simulink model "variense_block"  (R2018b)
settings: Solver=FixedStepDiscrete  StartTime=0.0  StopTime=inf  FixedStep=.0001  RelTol=1e-3
InitFcn:
  | addpath('..\ForceSensor\compile\release')
libraries: xpcutilitieslib x6, etargetslib x4, aerolibanimutils x1
settings Model: Creator=dds  LastModifiedBy=dds

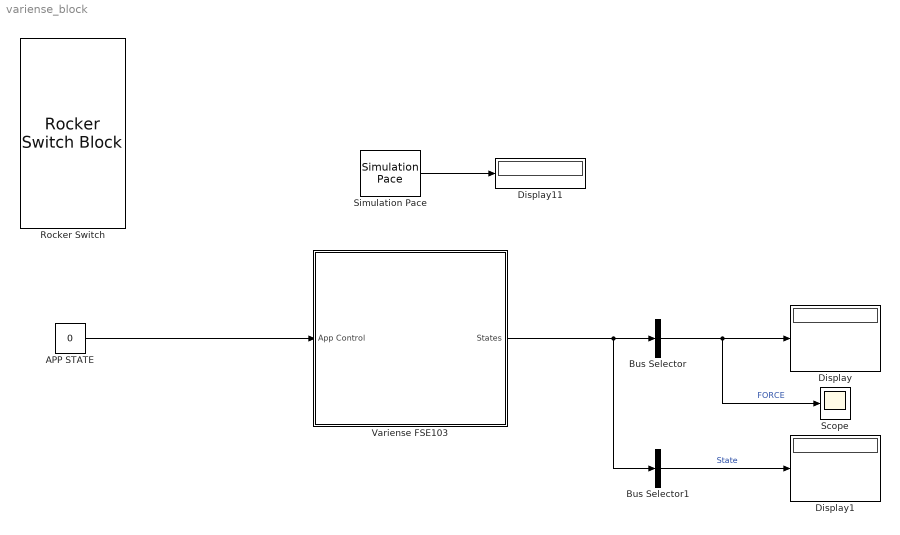
== system variense_block ==
  APP STATE : Constant  Value=0  OutDataTypeStr=uint32
  Bus Selector : BusSelector  OutputSignals=Fx,Fy,Fz  OutputAsBus=on
  Bus Selector1 : BusSelector  OutputSignals=Reception Rate [us],Packets received  OutputAsBus=on
  Display : Display
  Display1 : Display
  Display11 : Display
  Rocker Switch : RockerSwitchBlock  WebBlockId=99
      settings: Values={{'STOP', 'START'}, [1 0]}
  Scope : Scope
  Simulation Pace : aerolibanimutils/Simulation Pace  SimulationPace=1  SleepMode=Auto  OutputPaceError=on  SampleTime=-1
  "Variense FSE103 " : Subsystem  mask{id=1, port='COM8', baudrate=10.5Mbps, ts=1, reg_name='DefenceRobot', reg_size=512, st=0}
      mask prompts: id "Sensor Id"; ts "Sample Time [us]"; reg_name "Register Name"; reg_size "Register Size"; st "Start address"
      mask TypeOptions baudrate: 9600 btps | 57600 bps | 115200 bps | 1 Mbps | 2 Mbps | 3 Mbps | 4 Mbps | 4.5 Mbps | 10.5Mbps
      mask DialogControl DescGroupVar Prompt: IApp based Block
      mask DialogControl Container4 Prompt: Device Control Parameters
      mask DialogControl Container6 Prompt: Main Register Parameters
      mask Display:
      | image('variense.jpg')
      | color('red');
      | 
      | port_label('output', 1, 'Sensors' )
      | color('blue');
      | port_label('input', 1, 'App Control')
  wires:
  Simulation Pace/1 -> Display11/1
  APP STATE/1 -> "Variense FSE103 "/1(App Control)
  "Variense FSE103 "/1(States) -> Bus Selector1/1, Bus Selector/1
  Bus Selector/1 -> Scope/1, Display/1  "FORCE"
  Bus Selector1/1 -> Display1/1  "State"

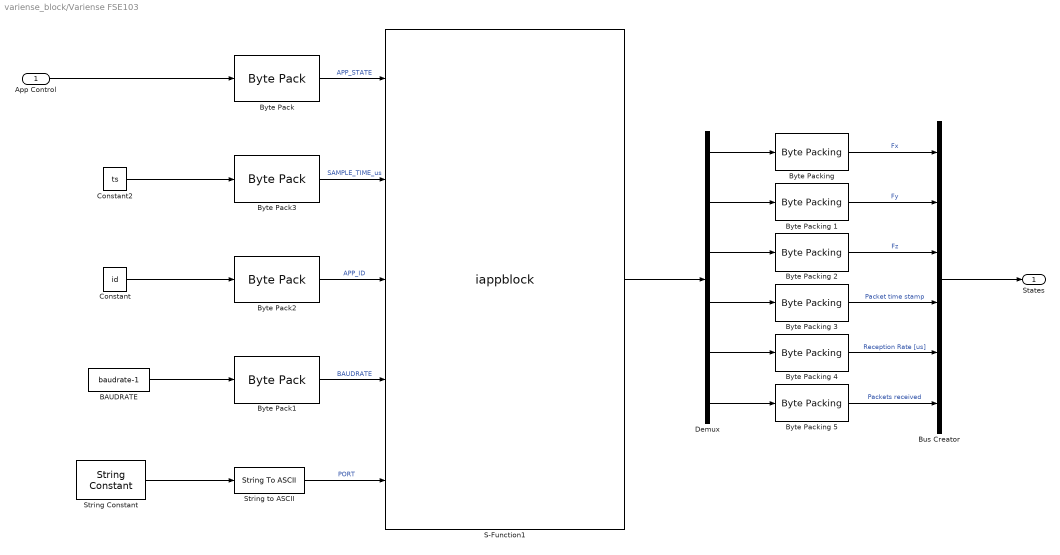
== system variense_block/Variense FSE103  ==
  App Control : Inport
  BAUDRATE : Constant  Value=baudrate-1  OutDataTypeStr=uint32
  Bus Creator : BusCreator  Inputs=6
  Byte Pack{,1..3} (4 alike) : etargetslib/Byte Pack  datatypes={'uint32'}  byteAlign=1
  Byte Packing {,1..5} (6 alike) : xpcutilitieslib/Byte Packing 
  Constant : Constant  Value=id  OutDataTypeStr=uint32
  Constant2 : Constant  Value=ts  OutDataTypeStr=uint32
  Demux : Demux  Outputs=6
  S-Function1 : S-Function  FunctionName=iappblock  Parameters=configText,prog,ts,trig,cmd  SFunctionDeploymentMode=off  EnableBusSupport=off  mask{configText=|, prog=which('ForceSensor.exe'), ts=-1, trig=off, cmd=off}
      mask configText=|
      | sprintf(['REGISTER_NAME  = %s' newline...
      |     'REGISTER_SIZE  = %i'            newline...
      |     'APP_STATE      =[%i,4 ,1, 1]'   newline...
      |     'SAMPLE_TIME_us =[%i,4 ,1, %i]'  newline...
      |     'APP_ID         =[%i,4 ,1, %i]'  newline...
      |     'BAUDRATE       =[%i,4 ,1, %i]'  newline...
      |     'PORT           =[%i,8 ,1, %s]'  newline...
      |     'SENSOR_OUTPUTS	=[%i,24,2,0 0 0 0]'   newline...
      |     ],reg_name,reg_size,st,st+4,ts,st+8,id,st+12,baudrate,st+16,port,st+24)
      mask prompts: configText "configuration Text"; prog "Program"; ts "Sample Time"; trig "Trigger enable"; cmd "Show console window"
  String Constant : StringConstant  String=port
  String to ASCII : StringToASCII  MaximumLength=8
  States : Outport
  wires:
  Constant2/1 -> Byte Pack3/1
  Constant/1 -> Byte Pack2/1
  String Constant/1 -> String to ASCII/1
  String to ASCII/1 -> S-Function1/5  "PORT"
  BAUDRATE/1 -> Byte Pack1/1
  App Control/1 -> Byte Pack/1
  Byte Pack2/1 -> S-Function1/3  "APP_ID"
  Byte Pack1/1 -> S-Function1/4  "BAUDRATE"
  Byte Pack3/1 -> S-Function1/2  "SAMPLE_TIME_us"
  Byte Pack/1 -> S-Function1/1  "APP_STATE"
  Bus Creator/1 -> States/1
  Byte Packing 2/1 -> Bus Creator/3  "Fz"
  Demux/2 -> Byte Packing 1/1
  Byte Packing 4/1 -> Bus Creator/5  "Reception Rate [us]"
  Byte Packing 5/1 -> Bus Creator/6  "Packets received"
  Byte Packing 1/1 -> Bus Creator/2  "Fy"
  "Byte Packing "/1 -> Bus Creator/1  "Fx"
  Demux/1 -> "Byte Packing "/1
  Demux/6 -> Byte Packing 5/1
  Byte Packing 3/1 -> Bus Creator/4  "Packet time stamp"
  Demux/5 -> Byte Packing 4/1
  S-Function1/1 -> Demux/1
  Demux/3 -> Byte Packing 2/1
  Demux/4 -> Byte Packing 3/1
